simulink model "gm_trans_123_alphabeta_dq_V1"  (R2022a)
settings: Solver=FixedStepDiscrete  StartTime=0.0  StopTime=0.2  RelTol=1e-3
InitFcn:
  | Ts_xadc = 0.1;
libraries: hdlmdlgenlib x6, simulink x4
settings Model: Creator=trichte  LastModifiedBy=Andre Merx
settings SolverCC: AlgebraicLoopSolver=TrustRegion
settings DataIOCC: LimitDataPoints=on  SaveFormat=Array  SaveOutput=off  SaveTime=off  ReturnWorkspaceOutputs=off
settings OptimizationCC: BlockReduction=off  ConditionallyExecuteInputs=off  DefaultParameterBehavior=Inlined  LifeSpan=inf
settings DebuggingCC: AlgebraicLoopMsg=error  SolverPrmCheckMsg=warning  InheritedTsInSrcMsg=none  SingleTaskRateTransMsg=error  UnconnectedInputMsg=warning  UnconnectedOutputMsg=warning  UnconnectedLineMsg=warning  AllowSymbolicDim=off  StrictBusMsg=ErrorOnBusTreatedAsVector  SFUnexpectedBacktrackingDiag=warning  SFNoUnconditionalDefaultTransitionDiag=warning  SFExecutionAtInitializationDiag=none  SFMachineParentedDataDiag=warning  ArithmeticOperatorsInVariantConditions=warning
settings HardwareCC: ProdBitPerPointer=32  ProdBitPerSizeT=32  ProdBitPerPtrDiffT=32  ProdLargestAtomicFloat=None  ProdIntDivRoundTo=Undefined  ProdEndianess=Unspecified  ProdWordSize=32  ProdHWDeviceType=ASIC/FPGA->ASIC/FPGA  ProdEqTarget=off
settings ModelReferenceCC: PropagateSignalLabelsOutOfModel=off
settings SFSimCC: SimUseLocalCustomCode=off  CustomCodeUndefinedFunction=UseInterfaceOnly
settings RTWCC: RTWUseLocalCustomCode=off
settings CodeAppCC: StateflowObjectComments=on
settings GRTTargetCC: TargetLangStandard=C89/C90 (ANSI)
settings ConfigComp: CovMetricSettings=dw  CovSaveCumulativeToWorkspaceVar=on  CovSaveSingleToWorkspaceVar=on  CovExternalEMLEnable=off  CovSFcnEnable=off

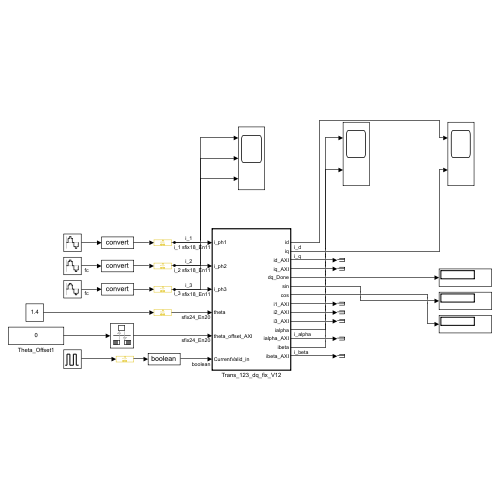
[thumbnail: Simulink's stored preview of the top-level diagram]
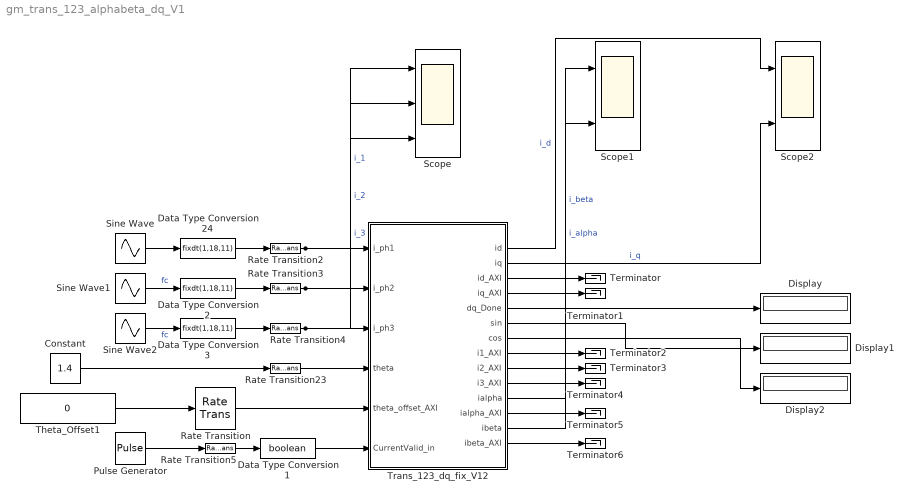
== system gm_trans_123_alphabeta_dq_V1 ==
  Constant : Constant  Value=1.4  OutDataTypeStr=fixdt(1,24,20)
  Data Type Conversion1 : DataTypeConversion  OutDataTypeStr=boolean  SaturateOnIntegerOverflow=off  RndMeth=Floor
  Data Type Conversion2 : DataTypeConversion  OutDataTypeStr=fixdt(1,18,11)  SaturateOnIntegerOverflow=off  RndMeth=Floor
  Data Type Conversion24 : DataTypeConversion  OutDataTypeStr=fixdt(1,18,11)  SaturateOnIntegerOverflow=off  RndMeth=Floor
  Data Type Conversion3 : DataTypeConversion  OutDataTypeStr=fixdt(1,18,11)  SaturateOnIntegerOverflow=off  RndMeth=Floor
  Display : Display
  Display1 : Display
  Display2 : Display
  Pulse Generator : DiscretePulseGenerator  PulseType=Time based  Period=1/100000  PulseWidth=5
  Rate Transition{,2..5,23} (6 alike) : RateTransition  OutPortSampleTime=T_50MHz
  Scope : Scope  NumInputPorts=3
  Scope1 : Scope  NumInputPorts=2
  Scope2 : Scope  NumInputPorts=2
  Sine Wave : Sin  Frequency=100  SampleTime=1/100000
  Sine Wave1 : Sin  Frequency=100  Phase=(2/3)*pi  SampleTime=1/100000
  Sine Wave2 : Sin  Frequency=100  Phase=(4/3)*pi  SampleTime=1/100000
  Terminator{,1..6} (7 alike) : Terminator
  Theta_Offset1 : Constant  Value=0  OutDataTypeStr=fixdt(1,24,20)
  Trans_123_dq_fix_V12 : Subsystem  TreatAsAtomicUnit=on
  wires:
  Sine Wave1/1 -> Data Type Conversion2/1  "fc"
  Data Type Conversion3/1 -> Rate Transition4/1
  Data Type Conversion2/1 -> Rate Transition3/1
  Data Type Conversion24/1 -> Rate Transition2/1
  Sine Wave/1 -> Data Type Conversion24/1
  Trans_123_dq_fix_V12/12(ialpha_AXI) -> Terminator5/1
  Trans_123_dq_fix_V12/6(sin) -> Display1/1
  Trans_123_dq_fix_V12/2(iq) -> Scope2/2  "i_q"
  Rate Transition5/1 -> Data Type Conversion1/1
  Trans_123_dq_fix_V12/10(i3_AXI) -> Terminator4/1
  Trans_123_dq_fix_V12/11(ialpha) -> Scope1/1  "i_alpha"
  Trans_123_dq_fix_V12/14(ibeta_AXI) -> Terminator6/1
  Constant/1 -> Rate Transition23/1
  Trans_123_dq_fix_V12/7(cos) -> Display2/1
  Trans_123_dq_fix_V12/4(iq_AXI) -> Terminator1/1
  Rate Transition23/1 -> Trans_123_dq_fix_V12/4(theta)
  Trans_123_dq_fix_V12/9(i2_AXI) -> Terminator3/1
  Pulse Generator/1 -> Rate Transition5/1
  Rate Transition4/1 -> Trans_123_dq_fix_V12/3(i_ph3), Scope/3  "i_3"
  Data Type Conversion1/1 -> Trans_123_dq_fix_V12/6(CurrentValid_in)
  Rate Transition/1 -> Trans_123_dq_fix_V12/5(theta_offset_AXI)
  Rate Transition2/1 -> Trans_123_dq_fix_V12/1(i_ph1), Scope/1  "i_1"
  Rate Transition3/1 -> Trans_123_dq_fix_V12/2(i_ph2), Scope/2  "i_2"
  Theta_Offset1/1 -> Rate Transition/1
  Trans_123_dq_fix_V12/1(id) -> Scope2/1  "i_d"
  Trans_123_dq_fix_V12/8(i1_AXI) -> Terminator2/1
  Trans_123_dq_fix_V12/5(dq_Done) -> Display/1
  Trans_123_dq_fix_V12/3(id_AXI) -> Terminator/1
  Trans_123_dq_fix_V12/13(ibeta) -> Scope1/2  "i_beta"
  Sine Wave2/1 -> Data Type Conversion3/1  "fc"

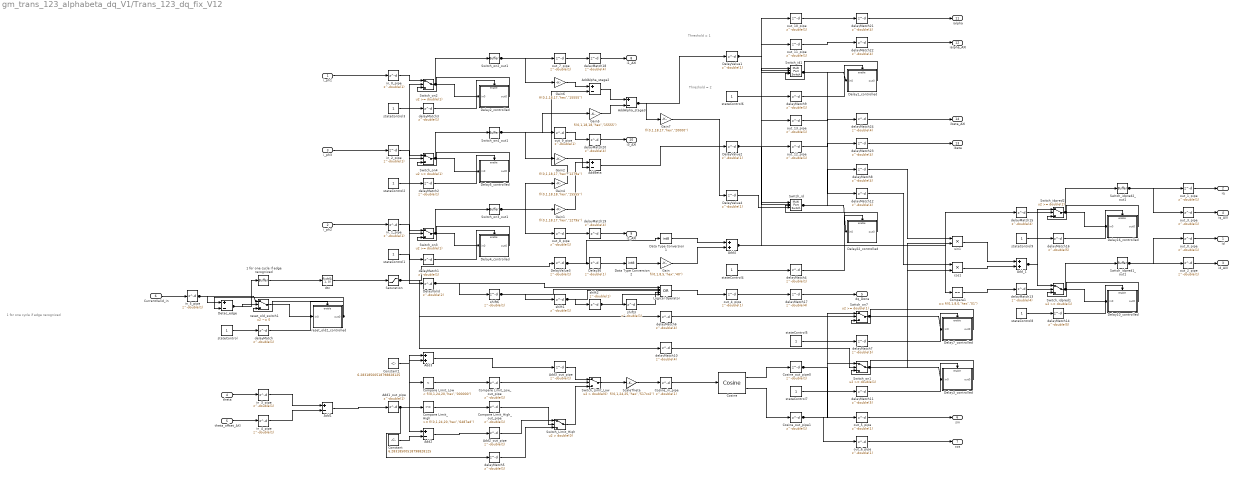
== system gm_trans_123_alphabeta_dq_V1/Trans_123_dq_fix_V12 ==
  note: Threshold = 2
  note: Threshold = 1
  note: 1 for one cycle if edge recognized
  i_ph1 : Inport  OutDataTypeStr=fixdt(1, 18, 11)  PortDimensions=1  SampleTime=2e-08
  i_ph2 : Inport  Port=2  OutDataTypeStr=fixdt(1, 18, 11)  PortDimensions=1  SampleTime=2e-08
  i_ph3 : Inport  Port=3  OutDataTypeStr=fixdt(1, 18, 11)  PortDimensions=1  SampleTime=2e-08
  theta : Inport  Port=4  OutDataTypeStr=fixdt(1, 24, 20)  PortDimensions=1  SampleTime=2e-08
  theta_offset_AXI : Inport  Port=5  OutDataTypeStr=fixdt(1, 24, 20)  PortDimensions=1  SampleTime=2e-08
  CurrentValid_in : Inport  Port=6  OutDataTypeStr=boolean  PortDimensions=1  SampleTime=2e-08
  1 for one cycle if edge recognized : hdlmdlgenlib/Buffer
      settings: SourceProductBaseCode=SL
  Add1 : Sum  Inputs=+-  AccumDataTypeStr=fixdt(1, 24, 20)  OutDataTypeStr=fixdt(1, 24, 20)  SampleTime=2e-08
  Add1_out_pipe : Delay  DelayLength=double(1)  InitialCondition=0  SampleTime=2e-08
  Add2 : Sum  Inputs=+-  AccumDataTypeStr=fixdt(1, 24, 20)  OutDataTypeStr=fixdt(1, 24, 20)  SampleTime=2e-08
  Add2_out_pipe : Delay  DelayLength=double(1)  InitialCondition=0  SampleTime=2e-08
  Add3 : Sum  AccumDataTypeStr=fixdt(1, 24, 20)  OutDataTypeStr=fixdt(1, 24, 20)  SampleTime=2e-08
  Add3_out_pipe : Delay  DelayLength=double(1)  InitialCondition=0  SampleTime=2e-08
  Add4 : Sum  AccumDataTypeStr=int8  OutDataTypeStr=int8  RndMeth=Simplest  SampleTime=2e-08
  AddAlpha_stage2 : Sum  Inputs=+-  AccumDataTypeStr=fixdt(1, 18, 11)  OutDataTypeStr=fixdt(1, 18, 11)  SampleTime=2e-08
  AddAlpha_stage3 : Sum  Inputs=+-  AccumDataTypeStr=fixdt(1, 18, 11)  OutDataTypeStr=fixdt(1, 18, 11)  SampleTime=2e-08
  AddBeta : Sum  Inputs=+-  AccumDataTypeStr=fixdt(1, 18, 11)  OutDataTypeStr=fixdt(1, 18, 11)  SampleTime=2e-08
  Add_1 : Sum  AccumDataTypeStr=fixdt(1, 18, 11)  OutDataTypeStr=fixdt(1, 18, 11)  SampleTime=2e-08
  Compare Limit_High : simulink/Logic and Bit Operations/Compare To Constant  relop=>=  const="fi(0,1,24,20,\"hex\",\"6487ed\")"  OutDataTypeStr=boolean
  Compare Limit_High_out_pipe : Delay  DelayLength=double(1)  InitialCondition=0  SampleTime=2e-08
  Compare Limit_Low : simulink/Logic and Bit Operations/Compare To Constant  relop=<  const="fi(0,1,24,20,\"hex\",\"000000\")"  OutDataTypeStr=boolean
  Compare Limit_Low_out_pipe : Delay  DelayLength=double(1)  InitialCondition=0  SampleTime=2e-08
  Compare1 : simulink/Logic and Bit Operations/Compare To Constant  relop===  const="fi(0,1,8,0,\"hex\",\"01\")"  OutDataTypeStr=boolean
  Constant : Constant  Value=6.28318500518798828125  OutDataTypeStr=fixdt(1, 24, 20)  SampleTime=2e-08
  Constant1 : Constant  Value=6.28318500518798828125  OutDataTypeStr=fixdt(1, 24, 20)  SampleTime=2e-08
  Cosine : simulink/Lookup Tables/Cosine  Formula=sin(2*pi*u) and cos(2*pi*u)  NumDataPoints=(2^9)+1  OutputWordLength=16  InternalRulePriority=Precision
      settings: SourceProductBaseCode=SL
  Cosine_in_pipe : Delay  DelayLength=double(1)  InitialCondition=0  SampleTime=2e-08
  Cosine_out_pipe0 : Delay  DelayLength=double(1)  InitialCondition=0  SampleTime=2e-08
  Cosine_out_pipe1 : Delay  DelayLength=double(1)  InitialCondition=0  SampleTime=2e-08
  Data Type Conversion1 : DataTypeConversion  OutDataTypeStr=int8  SampleTime=2e-08  SaturateOnIntegerOverflow=off  RndMeth=Floor
  Data Type Conversion2 : DataTypeConversion  OutDataTypeStr=int8  SampleTime=2e-08  SaturateOnIntegerOverflow=off  RndMeth=Floor
  Delay10_controlled : Subsystem
  Delay16_controlled : Subsystem
  Delay1_controlled : Subsystem
  Delay22_controlled : Subsystem
  Delay2_controlled : Subsystem
  Delay36 : Delay  DelayLength=double(1)  InitialCondition=0  SampleTime=2e-08
  Delay3_controlled : Subsystem
  Delay4_controlled : Subsystem
  Delay5_controlled : Subsystem
  Delay7_controlled : Subsystem
  DelayValid : Delay  DelayLength=double(2)  InitialCondition=0  SampleTime=2e-08
  DelayValue{1..4} (4 alike) : Delay  DelayLength=double(1)  InitialCondition=0  SampleTime=2e-08
  Detec_edge : Sum  Inputs=+-  AccumDataTypeStr=int8  OutDataTypeStr=int8  SampleTime=2e-08
  Gain : Gain  Gain="fi(0,1,8,5,\"hex\",\"40\")"  ParamDataTypeStr=fixdt(1, 8, 5)  OutDataTypeStr=fixdt(1, 16, 5)  RndMeth=Simplest  SampleTime=2e-08
  Gain1 : Gain  Gain="fi(0,1,18,17,\"hex\",\"1279a\")"  ParamDataTypeStr=fixdt(1, 18, 17)  OutDataTypeStr=fixdt(1, 18, 11)  SampleTime=2e-08
  Gain2 : Gain  Gain="fi(0,1,18,17,\"hex\",\"1279a\")"  ParamDataTypeStr=fixdt(1, 18, 17)  OutDataTypeStr=fixdt(1, 18, 11)  SampleTime=2e-08
  Gain4 : Gain  Gain="fi(0,1,18,18,\"hex\",\"15555\")"  ParamDataTypeStr=fixdt(1, 18, 18)  OutDataTypeStr=fixdt(1, 18, 11)  SampleTime=2e-08
  Gain5 : Gain  Gain="fi(0,1,18,18,\"hex\",\"15555\")"  ParamDataTypeStr=fixdt(1, 18, 18)  OutDataTypeStr=fixdt(1, 18, 11)  SampleTime=2e-08
  Gain6 : Gain  Gain="fi(0,1,18,17,\"hex\",\"15555\")"  ParamDataTypeStr=fixdt(1, 18, 17)  OutDataTypeStr=fixdt(1, 18, 11)  SampleTime=2e-08
  Gain7 : Gain  Gain="fi(0,1,18,17,\"hex\",\"20000\")"  ParamDataTypeStr=fixdt(1, 18, 17)  OutDataTypeStr=fixdt(1, 18, 11)  SampleTime=2e-08
  Logical Operator : Logic  Operator=OR  Inputs=5  AllPortsSameDT=off  OutDataTypeStr=boolean  SampleTime=2e-08
  Saturation : Saturate  UpperLimit="fi(0,0,1,0,\"hex\",\"1\")"  LowerLimit="fi(0,0,1,0,\"hex\",\"0\")"  SampleTime=2e-08  OutDataTypeStr=fixdt(0, 1, 0)
  ScaleTheta : Gain  Gain="fi(0,1,24,25,\"hex\",\"517cc2\")"  ParamDataTypeStr=fixdt(1, 24, 25)  OutDataTypeStr=fixdt(1, 24, 20)  SampleTime=2e-08
  Switch_Limit_High : Switch  Criteria=u2 > Threshold  Threshold=double(0)  OutDataTypeStr=fixdt(1, 24, 20)  SampleTime=2e-08  SaturateOnIntegerOverflow=off  InputSameDT=off
  Switch_Limit_Low : Switch  Criteria=u2 > Threshold  Threshold=double(0)  OutDataTypeStr=fixdt(1, 24, 20)  SampleTime=2e-08  SaturateOnIntegerOverflow=off  InputSameDT=off
  Switch_id : MultiPortSwitch  Inputs=2  DataPortForDefault=Additional data port  DiagnosticForDefault=None  OutDataTypeStr=fixdt(1, 18, 11)  RndMeth=Simplest  SampleTime=2e-08  SaturateOnIntegerOverflow=off  InputSameDT=off
  Switch_id1 : MultiPortSwitch  Inputs=2  DataPortForDefault=Additional data port  DiagnosticForDefault=None  OutDataTypeStr=fixdt(1, 18, 11)  RndMeth=Simplest  SampleTime=2e-08  SaturateOnIntegerOverflow=off  InputSameDT=off
  Switch_idpred1 : Switch  Threshold=double(1)  OutDataTypeStr=fixdt(1, 18, 11)  RndMeth=Simplest  SampleTime=2e-08  SaturateOnIntegerOverflow=off  InputSameDT=off
  Switch_idpred1_out1 : hdlmdlgenlib/Buffer
      settings: SourceProductBaseCode=SL
  Switch_idpred2 : Switch  Threshold=double(2)  OutDataTypeStr=fixdt(1, 18, 11)  RndMeth=Simplest  SampleTime=2e-08  SaturateOnIntegerOverflow=off  InputSameDT=off
  Switch_idpred2_out1 : hdlmdlgenlib/Buffer
      settings: SourceProductBaseCode=SL
  Switch_on1 : Switch  Threshold=double(1)  OutDataTypeStr=fixdt(1, 16, 14)  SampleTime=2e-08  SaturateOnIntegerOverflow=off  InputSameDT=off
  Switch_on2 : Switch  Threshold=double(1)  OutDataTypeStr=fixdt(1, 18, 11)  RndMeth=Simplest  SampleTime=2e-08  SaturateOnIntegerOverflow=off  InputSameDT=off
  Switch_on2_out1 : hdlmdlgenlib/Buffer
      settings: SourceProductBaseCode=SL
  Switch_on3 : Switch  Threshold=double(1)  OutDataTypeStr=fixdt(1, 18, 11)  RndMeth=Simplest  SampleTime=2e-08  SaturateOnIntegerOverflow=off  InputSameDT=off
  Switch_on3_out1 : hdlmdlgenlib/Buffer
      settings: SourceProductBaseCode=SL
  Switch_on4 : Switch  Threshold=double(1)  OutDataTypeStr=fixdt(1, 18, 11)  RndMeth=Simplest  SampleTime=2e-08  SaturateOnIntegerOverflow=off  InputSameDT=off
  Switch_on4_out1 : hdlmdlgenlib/Buffer
      settings: SourceProductBaseCode=SL
  Switch_on7 : Switch  Threshold=double(1)  OutDataTypeStr=fixdt(1, 16, 14)  SampleTime=2e-08  SaturateOnIntegerOverflow=off  InputSameDT=off
  cos1 : Product  Inputs=**  OutDataTypeStr=fixdt(1, 18, 11)  RndMeth=Simplest  SampleTime=2e-08
  delayMatch{,1..5,9} (7 alike) : Delay  DelayLength=double(1)  InitialCondition=0  SampleTime=2e-08
  delayMatch{6,8,10,12..13,15,17..24} (14 alike) : Delay  DelayLength=double(4)  InitialCondition=0  SampleTime=2e-08
  delayMatch{7,11,14,16} (4 alike) : Delay  DelayLength=double(5)  InitialCondition=0  SampleTime=2e-08
  dtc : DataTypeConversion  OutDataTypeStr=fixdt(0, 1, 0)  SampleTime=2e-08  RndMeth=Floor
  in_0_pipe : Delay  DelayLength=double(1)  InitialCondition=0  SampleTime=2e-08
  in_1_pipe : Delay  DelayLength=double(1)  InitialCondition=0  SampleTime=2e-08
  in_2_pipe : Delay  DelayLength=double(1)  InitialCondition=0  SampleTime=2e-08
  in_3_pipe : Delay  DelayLength=double(1)  InitialCondition=0  SampleTime=2e-08
  in_4_pipe : Delay  DelayLength=double(1)  InitialCondition=0  SampleTime=2e-08
  in_5_pipe : Delay  DelayLength=double(1)  InitialCondition=0  SampleTime=2e-08
  out_0_pipe : Delay  DelayLength=double(1)  InitialCondition=0  SampleTime=2e-08
  out_10_pipe : Delay  DelayLength=double(1)  InitialCondition=0  SampleTime=2e-08
  out_11_pipe : Delay  DelayLength=double(1)  InitialCondition=0  SampleTime=2e-08
  out_12_pipe : Delay  DelayLength=double(1)  InitialCondition=0  SampleTime=2e-08
  out_13_pipe : Delay  DelayLength=double(1)  InitialCondition=0  SampleTime=2e-08
  out_1_pipe : Delay  DelayLength=double(1)  InitialCondition=0  SampleTime=2e-08
  out_2_pipe : Delay  DelayLength=double(1)  InitialCondition=0  SampleTime=2e-08
  out_3_pipe : Delay  DelayLength=double(1)  InitialCondition=0  SampleTime=2e-08
  out_4_pipe : Delay  DelayLength=double(1)  InitialCondition=0  SampleTime=2e-08
  out_5_pipe : Delay  DelayLength=double(1)  InitialCondition=0  SampleTime=2e-08
  out_6_pipe : Delay  DelayLength=double(1)  InitialCondition=0  SampleTime=2e-08
  out_7_pipe : Delay  DelayLength=double(1)  InitialCondition=0  SampleTime=2e-08
  out_8_pipe : Delay  DelayLength=double(1)  InitialCondition=0  SampleTime=2e-08
  out_9_pipe : Delay  DelayLength=double(1)  InitialCondition=0  SampleTime=2e-08
  reset_old2_controlled : Subsystem
  reset_old_switch1 : Switch  Criteria=u2 ~= 0  Threshold=double(0)  OutDataTypeStr=boolean  SampleTime=2e-08  SaturateOnIntegerOverflow=off  InputSameDT=off
  shift{1..3,6} (4 alike) : Delay  DelayLength=double(1)  InitialCondition=0  SampleTime=2e-08
  sin1 : Product  Inputs=**  OutDataTypeStr=fixdt(1, 18, 11)  RndMeth=Simplest  SampleTime=2e-08
  stateControl{,1..9} (10 alike) : Constant  OutDataTypeStr=boolean  SampleTime=2e-08
  id : Outport  SampleTime=2e-08  VectorParamsAs1DForOutWhenUnconnected=off
  iq : Outport  Port=2  SampleTime=2e-08  VectorParamsAs1DForOutWhenUnconnected=off
  id_AXI : Outport  Port=3  SampleTime=2e-08  VectorParamsAs1DForOutWhenUnconnected=off
  iq_AXI : Outport  Port=4  SampleTime=2e-08  VectorParamsAs1DForOutWhenUnconnected=off
  dq_Done : Outport  Port=5  SampleTime=2e-08  VectorParamsAs1DForOutWhenUnconnected=off
  sin : Outport  Port=6  SampleTime=2e-08  VectorParamsAs1DForOutWhenUnconnected=off
  cos : Outport  Port=7  SampleTime=2e-08  VectorParamsAs1DForOutWhenUnconnected=off
  i1_AXI : Outport  Port=8  SampleTime=2e-08  VectorParamsAs1DForOutWhenUnconnected=off
  i2_AXI : Outport  Port=9  SampleTime=2e-08  VectorParamsAs1DForOutWhenUnconnected=off
  i3_AXI : Outport  Port=10  SampleTime=2e-08  VectorParamsAs1DForOutWhenUnconnected=off
  ialpha : Outport  Port=11  SampleTime=2e-08  VectorParamsAs1DForOutWhenUnconnected=off
  ialpha_AXI : Outport  Port=12  SampleTime=2e-08  VectorParamsAs1DForOutWhenUnconnected=off
  ibeta : Outport  Port=13  SampleTime=2e-08  VectorParamsAs1DForOutWhenUnconnected=off
  ibeta_AXI : Outport  Port=14  SampleTime=2e-08  VectorParamsAs1DForOutWhenUnconnected=off
  wires:
  in_0_pipe/1 -> Switch_on2/1
  in_1_pipe/1 -> Switch_on3/1
  in_2_pipe/1 -> Switch_on4/1
  in_3_pipe/1 -> Add1/1
  in_4_pipe/1 -> Add1/2
  in_5_pipe/1 -> reset_old_switch1/1, Detec_edge/1
  delayMatch5/1 -> Switch_Limit_High/3
  Add2_out_pipe/1 -> Switch_Limit_High/1
  Add3_out_pipe/1 -> Switch_Limit_Low/1
  delayMatch15/1 -> Switch_idpred2/2
  AddAlpha_stage3/1 -> Gain7/1, DelayValue1/1
  AddBeta/1 -> DelayValue2/1
  Add_1/1 -> Switch_idpred1/1, Switch_idpred2/1
  Compare Limit_High_out_pipe/1 -> Switch_Limit_High/2
  Compare Limit_Low_out_pipe/1 -> Switch_Limit_Low/2
  delayMatch13/1 -> Switch_idpred1/2
  Constant/1 -> Add2/2
  Constant1/1 -> Add3/2
  Cosine_out_pipe0/1 -> out_5_pipe/1, Switch_on7/1
  Cosine_out_pipe1/1 -> out_6_pipe/1, Switch_on1/1
  Data Type Conversion1/1 -> Add4/1
  Data Type Conversion2/1 -> Gain/1
  Delay36/1 -> Data Type Conversion2/1
  DelayValid/1 -> Logical Operator/1, shift6/1
  DelayValue1/1 -> out_11_pipe/1, out_10_pipe/1, Switch_id1/2
  DelayValue2/1 -> out_13_pipe/1, out_12_pipe/1, Switch_id/2, Switch_id1/3
  DelayValue3/1 -> Data Type Conversion1/1, Delay36/1
  DelayValue4/1 -> Switch_id/3
  1 for one cycle if edge recognized/1 -> dtc/1
  Gain/1 -> Add4/2
  Gain1/1 -> AddBeta/1
  Gain2/1 -> AddBeta/2
  Gain4/1 -> AddAlpha_stage2/2
  Gain5/1 -> AddAlpha_stage3/2
  Gain6/1 -> AddAlpha_stage2/1
  Gain7/1 -> DelayValue4/1
  Logical Operator/1 -> out_4_pipe/1
  delayMatch6/1 -> Switch_on7/2
  ScaleTheta/1 -> Cosine_in_pipe/1
  Switch_Limit_High/1 -> Switch_Limit_Low/3
  Switch_Limit_Low/1 -> ScaleTheta/1
  delayMatch8/1 -> sin1/1
  delayMatch12/1 -> cos1/1
  Switch_idpred1_out1/1 -> out_2_pipe/1, out_0_pipe/1
  Switch_idpred2_out1/1 -> out_3_pipe/1, out_1_pipe/1
  Switch_on2_out1/1 -> out_7_pipe/1, Gain6/1
  Switch_on3_out1/1 -> out_8_pipe/1, Gain4/1, Gain1/1
  Switch_on4_out1/1 -> out_9_pipe/1, Gain5/1, Gain2/1
  cos1/1 -> Add_1/2
  shift1/1 -> Logical Operator/3, shift2/1
  shift2/1 -> Logical Operator/4, shift3/1
  shift3/1 -> Logical Operator/5
  shift6/1 -> Logical Operator/2, shift1/1
  sin1/1 -> Add_1/1
  out_0_pipe/1 -> id/1
  out_1_pipe/1 -> iq/1
  out_2_pipe/1 -> id_AXI/1
  out_3_pipe/1 -> iq_AXI/1
  delayMatch17/1 -> dq_Done/1
  out_5_pipe/1 -> sin/1
  out_6_pipe/1 -> cos/1
  delayMatch18/1 -> i1_AXI/1
  delayMatch19/1 -> i2_AXI/1
  delayMatch20/1 -> i3_AXI/1
  delayMatch21/1 -> ialpha/1
  delayMatch22/1 -> ialpha_AXI/1
  delayMatch23/1 -> ibeta/1
  delayMatch24/1 -> ibeta_AXI/1
  Add1/1 -> Add1_out_pipe/1
  Add2/1 -> Add2_out_pipe/1
  Add3/1 -> Add3_out_pipe/1
  Compare Limit_High/1 -> Compare Limit_High_out_pipe/1
  Compare Limit_Low/1 -> Compare Limit_Low_out_pipe/1
  i_ph1/1 -> in_0_pipe/1
  i_ph2/1 -> in_1_pipe/1
  i_ph3/1 -> in_2_pipe/1
  theta/1 -> in_3_pipe/1
  theta_offset_AXI/1 -> in_4_pipe/1
  CurrentValid_in/1 -> in_5_pipe/1
  Cosine/1 -> Cosine_out_pipe0/1
  Cosine/2 -> Cosine_out_pipe1/1
  Cosine_in_pipe/1 -> Cosine/1
  AddAlpha_stage2/1 -> AddAlpha_stage3/1
  dtc/1 -> Saturation/1
  delayMatch/1 -> reset_old2_controlled/Enable
  delayMatch1/1 -> Delay4_controlled/Enable
  delayMatch2/1 -> Delay5_controlled/Enable
  delayMatch3/1 -> Delay2_controlled/Enable
  delayMatch4/1 -> Delay22_controlled/Enable
  delayMatch7/1 -> Delay7_controlled/Enable
  delayMatch9/1 -> Delay1_controlled/Enable
  delayMatch11/1 -> Delay3_controlled/Enable
  delayMatch14/1 -> Delay10_controlled/Enable
  delayMatch16/1 -> Delay16_controlled/Enable
  stateControl/1 -> delayMatch/1
  stateControl1/1 -> delayMatch1/1
  stateControl2/1 -> delayMatch2/1
  stateControl3/1 -> delayMatch3/1
  stateControl4/1 -> delayMatch4/1
  Add1_out_pipe/1 -> delayMatch5/1, Compare Limit_Low/1, Compare Limit_High/1, Add3/1, Add2/1
  delayMatch10/1 -> Switch_on1/2
  stateControl5/1 -> delayMatch7/1
  stateControl6/1 -> delayMatch9/1
  Saturation/1 -> delayMatch10/1, delayMatch6/1, DelayValue3/1, DelayValid/1, Switch_on3/2, Switch_on4/2, Switch_on2/2
  stateControl7/1 -> delayMatch11/1
  Compare1/1 -> delayMatch13/1
  stateControl8/1 -> delayMatch14/1
  Add4/1 -> delayMatch15/1, Compare1/1, Switch_id/1, Switch_id1/1
  stateControl9/1 -> delayMatch16/1
  out_4_pipe/1 -> delayMatch17/1
  out_7_pipe/1 -> delayMatch18/1
  out_8_pipe/1 -> delayMatch19/1
  out_9_pipe/1 -> delayMatch20/1
  out_10_pipe/1 -> delayMatch21/1
  out_11_pipe/1 -> delayMatch22/1
  out_12_pipe/1 -> delayMatch23/1
  out_13_pipe/1 -> delayMatch24/1
  reset_old_switch1/1 -> reset_old2_controlled/1(in0)
  reset_old2_controlled/1(out0) -> reset_old_switch1/3, Detec_edge/2
  Detec_edge/1 -> 1 for one cycle if edge recognized/1, reset_old_switch1/2
  Delay4_controlled/1(out0) -> Switch_on3/3
  Switch_on3/1 -> Switch_on3_out1/1, Delay4_controlled/1(in0)
  Delay5_controlled/1(out0) -> Switch_on4/3
  Switch_on4/1 -> Switch_on4_out1/1, Delay5_controlled/1(in0)
  Delay2_controlled/1(out0) -> Switch_on2/3
  Switch_on2/1 -> Switch_on2_out1/1, Delay2_controlled/1(in0)
  Delay22_controlled/1(out0) -> Switch_id/4
  Switch_id/1 -> Delay22_controlled/1(in0), delayMatch8/1
  Delay7_controlled/1(out0) -> Switch_on7/3
  Switch_on7/1 -> Delay7_controlled/1(in0), sin1/2
  Delay1_controlled/1(out0) -> Switch_id1/4
  Switch_id1/1 -> Delay1_controlled/1(in0), delayMatch12/1
  Delay3_controlled/1(out0) -> Switch_on1/3
  Switch_on1/1 -> Delay3_controlled/1(in0), cos1/2
  Delay10_controlled/1(out0) -> Switch_idpred1/3
  Switch_idpred1/1 -> Switch_idpred1_out1/1, Delay10_controlled/1(in0)
  Delay16_controlled/1(out0) -> Switch_idpred2/3
  Switch_idpred2/1 -> Switch_idpred2_out1/1, Delay16_controlled/1(in0)

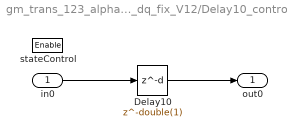
== system gm_trans_123_alphabeta_dq_V1/Trans_123_dq_fix_V12/Delay10_controlled ==
  in0 : Inport  OutDataTypeStr=fixdt(1, 18, 11)  SampleTime=2e-08
  stateControl : EnablePort  OutDataTypeStr=boolean
  Delay10 : Delay  DelayLength=double(1)  InitialCondition=0  SampleTime=2e-08
  out0 : Outport  OutDataTypeStr=fixdt(1, 18, 11)  SampleTime=2e-08
  wires:
  Delay10/1 -> out0/1
  in0/1 -> Delay10/1

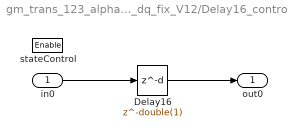
== system gm_trans_123_alphabeta_dq_V1/Trans_123_dq_fix_V12/Delay16_controlled ==
  in0 : Inport  OutDataTypeStr=fixdt(1, 18, 11)  SampleTime=2e-08
  stateControl : EnablePort  OutDataTypeStr=boolean
  Delay16 : Delay  DelayLength=double(1)  InitialCondition=0  SampleTime=2e-08
  out0 : Outport  OutDataTypeStr=fixdt(1, 18, 11)  SampleTime=2e-08
  wires:
  Delay16/1 -> out0/1
  in0/1 -> Delay16/1

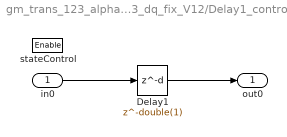
== system gm_trans_123_alphabeta_dq_V1/Trans_123_dq_fix_V12/Delay1_controlled ==
  in0 : Inport  OutDataTypeStr=fixdt(1, 18, 11)  SampleTime=2e-08
  stateControl : EnablePort  OutDataTypeStr=boolean
  Delay1 : Delay  DelayLength=double(1)  InitialCondition=0  SampleTime=2e-08
  out0 : Outport  OutDataTypeStr=fixdt(1, 18, 11)  SampleTime=2e-08
  wires:
  Delay1/1 -> out0/1
  in0/1 -> Delay1/1

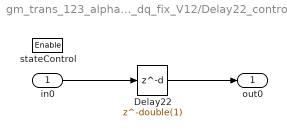
== system gm_trans_123_alphabeta_dq_V1/Trans_123_dq_fix_V12/Delay22_controlled ==
  in0 : Inport  OutDataTypeStr=fixdt(1, 18, 11)  SampleTime=2e-08
  stateControl : EnablePort  OutDataTypeStr=boolean
  Delay22 : Delay  DelayLength=double(1)  InitialCondition=0  SampleTime=2e-08
  out0 : Outport  OutDataTypeStr=fixdt(1, 18, 11)  SampleTime=2e-08
  wires:
  Delay22/1 -> out0/1
  in0/1 -> Delay22/1

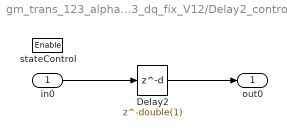
== system gm_trans_123_alphabeta_dq_V1/Trans_123_dq_fix_V12/Delay2_controlled ==
  in0 : Inport  OutDataTypeStr=fixdt(1, 18, 11)  SampleTime=2e-08
  stateControl : EnablePort  OutDataTypeStr=boolean
  Delay2 : Delay  DelayLength=double(1)  InitialCondition=0  SampleTime=2e-08
  out0 : Outport  OutDataTypeStr=fixdt(1, 18, 11)  SampleTime=2e-08
  wires:
  Delay2/1 -> out0/1
  in0/1 -> Delay2/1

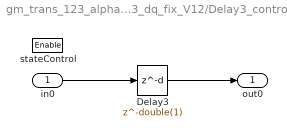
== system gm_trans_123_alphabeta_dq_V1/Trans_123_dq_fix_V12/Delay3_controlled ==
  in0 : Inport  OutDataTypeStr=fixdt(1, 16, 14)  SampleTime=2e-08
  stateControl : EnablePort  OutDataTypeStr=boolean
  Delay3 : Delay  DelayLength=double(1)  InitialCondition=0  SampleTime=2e-08
  out0 : Outport  OutDataTypeStr=fixdt(1, 16, 14)  SampleTime=2e-08
  wires:
  Delay3/1 -> out0/1
  in0/1 -> Delay3/1

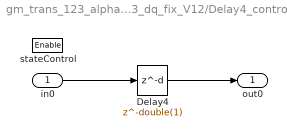
== system gm_trans_123_alphabeta_dq_V1/Trans_123_dq_fix_V12/Delay4_controlled ==
  in0 : Inport  OutDataTypeStr=fixdt(1, 18, 11)  SampleTime=2e-08
  stateControl : EnablePort  OutDataTypeStr=boolean
  Delay4 : Delay  DelayLength=double(1)  InitialCondition=0  SampleTime=2e-08
  out0 : Outport  OutDataTypeStr=fixdt(1, 18, 11)  SampleTime=2e-08
  wires:
  Delay4/1 -> out0/1
  in0/1 -> Delay4/1

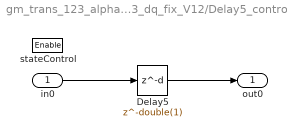
== system gm_trans_123_alphabeta_dq_V1/Trans_123_dq_fix_V12/Delay5_controlled ==
  in0 : Inport  OutDataTypeStr=fixdt(1, 18, 11)  SampleTime=2e-08
  stateControl : EnablePort  OutDataTypeStr=boolean
  Delay5 : Delay  DelayLength=double(1)  InitialCondition=0  SampleTime=2e-08
  out0 : Outport  OutDataTypeStr=fixdt(1, 18, 11)  SampleTime=2e-08
  wires:
  Delay5/1 -> out0/1
  in0/1 -> Delay5/1

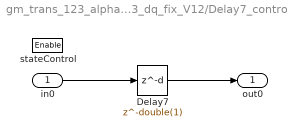
== system gm_trans_123_alphabeta_dq_V1/Trans_123_dq_fix_V12/Delay7_controlled ==
  in0 : Inport  OutDataTypeStr=fixdt(1, 16, 14)  SampleTime=2e-08
  stateControl : EnablePort  OutDataTypeStr=boolean
  Delay7 : Delay  DelayLength=double(1)  InitialCondition=0  SampleTime=2e-08
  out0 : Outport  OutDataTypeStr=fixdt(1, 16, 14)  SampleTime=2e-08
  wires:
  Delay7/1 -> out0/1
  in0/1 -> Delay7/1

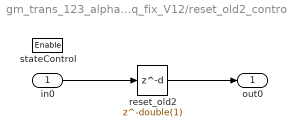
== system gm_trans_123_alphabeta_dq_V1/Trans_123_dq_fix_V12/reset_old2_controlled ==
  in0 : Inport  OutDataTypeStr=boolean  SampleTime=2e-08
  stateControl : EnablePort  OutDataTypeStr=boolean
  reset_old2 : Delay  DelayLength=double(1)  InitialCondition=0  SampleTime=2e-08
  out0 : Outport  OutDataTypeStr=boolean  SampleTime=2e-08
  wires:
  reset_old2/1 -> out0/1
  in0/1 -> reset_old2/1
